simulink model "demoProxyFRDM"  (R2016a)
settings: Solver=FixedStepAuto  StartTime=0.0  StopTime=inf  FixedStep=1  RelTol=1e-3
libraries: frdmKL25Z x2, frdmkl25zlib x1
settings Model: SimulationMode=external  ExtModeTrigDuration=5  Creator=user  LastModifiedBy=user
settings OptimizationCC: OptimizeModelRefInitCode=on  LifeSpan=1  MaxStackSize=64
settings HardwareCC: ProdBitPerPointer=32  ProdLargestAtomicInteger=Long  ProdLargestAtomicFloat=Double  ProdWordSize=32  ProdHWDeviceType=ARM Compatible->ARM Cortex
settings RTWCC: SystemTargetFile=ert.tlc  HardwareBoard=Freescale FRDM-KL25Z  TemplateMakefile=ert_default_tmf  GenerateReport=on  Toolchain=GNU Tools for ARM Embedded Processors  IncludeHyperlinkInReport=on  LaunchReport=on  GenerateTraceInfo=on  GenerateTraceReport=on  GenerateTraceReportSl=on  GenerateTraceReportSf=on  GenerateTraceReportEml=on
settings CodeAppCC: ForceParamTrailComments=on  IgnoreCustomStorageClasses=off  OperatorAnnotations=on  SimulinkDataObjDesc=on  SFDataObjDesc=on  MATLABFcnDesc=on  InsertBlockDesc=on  MATLABSourceComments=on

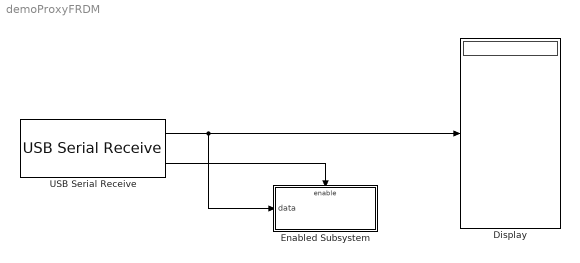
== system demoProxyFRDM ==
  Display : Display
  Enabled Subsystem : Subsystem  TreatAsAtomicUnit=on
  USB Serial Receive : frdmKL25Z/USB Serial Receive  msgLen=10  SimulateUsing=Code generation
  wires:
  USB Serial Receive/2 -> Enabled Subsystem/Enable
  USB Serial Receive/1 -> Enabled Subsystem/1(data), Display/1

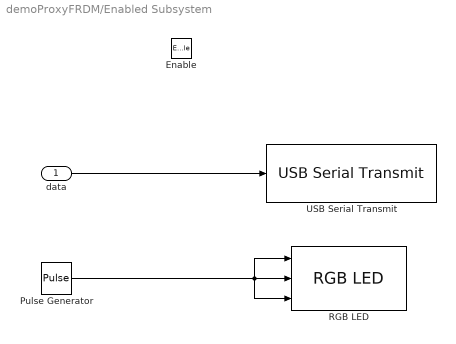
== system demoProxyFRDM/Enabled Subsystem ==
  data : Inport
  Enable : EnablePort
  Pulse Generator : DiscretePulseGenerator  Amplitude=100  SampleTime=-1
  RGB LED : frdmkl25zlib/RGB LED
  USB Serial Transmit : frdmKL25Z/USB Serial Transmit  SimulateUsing=Code generation
  wires:
  Pulse Generator/1 -> RGB LED/3, RGB LED/1, RGB LED/2
  data/1 -> USB Serial Transmit/1
